simulink model "Fig237"  (R2014b)
settings: Solver=ode3  StartTime=0.0  StopTime=10  FixedStep=2e-5  RelTol=1e-5
libraries: commfilt2 x1, commchan3 x1, commsink2 x1, commrandsrc2 x1
settings Model: Creator=Dennis Silage  LastModifiedBy=Silage
settings DataIOCC: SignalLoggingSaveFormat=ModelDataLogs
settings OptimizationCC: ExpressionDepthLimit=2147483647  InitFltsAndDblsToZero=on
settings DebuggingCC: UnderspecifiedInitializationDetection=Classic  MergeDetectMultiDrivingBlocksExec=none  SolverPrmCheckMsg=none  FcnCallInpInsideContextMsg=UseLocalSettings  StateNameClashWarn=warning
settings GRTTargetCC: CombineOutputUpdateFcns=off  GRTInterface=on

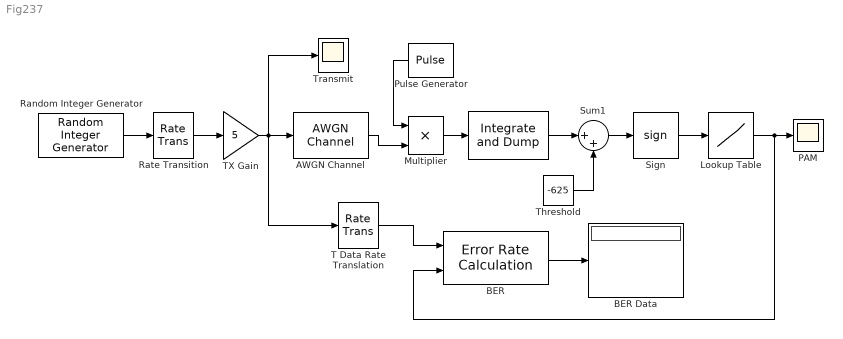
== system Fig237 ==
  " " : commfilt2/Integrate and Dump  obssamples=50  offsetsamples=0  nodump=off  roundingMode=Floor  overflowMode=off
  AWGN Channel : commchan3/AWGN Channel  InputProcessing=Inherited (this choice will be removed - see release notes)  seed=randseed  noiseMode="Signal to noise ratio  (Eb/No)"  EbNodB=40  EsNodB=10  SNRdB=10  bitsPerSym=1  Ps=25  Tsym=1e-3  variance=0
  BER : commsink2/Error Rate Calculation  N=1  st_delay=0  cp_mode=Entire frame  subframe=[]  PMode=Port  WsName=ErrorVec  RsMode2=off  stop=off  numErr=100  maxBits=1e6
  BER Data : Display
  Lookup Table : Lookup_n-D  NumberOfTableDimensions=1  BreakpointsForDimension1=[-1, 0, 1]  Table=[0, 0, 5]  InternalRulePriority=Speed  RndMeth=Nearest  InputSameDT=on
  Multiplier : Product  RndMeth=Zero
  PAM : Scope
      settings: TimeRange=0.05  YMin=-8  YMax=8
  Pulse Generator : DiscretePulseGenerator  PulseType=Time based  Amplitude=5  Period=1e-3  PulseWidth=98
  Random Integer Generator : commrandsrc2/Random Integer Generator  mul=2  seed=randseed  Ts=1e-3  frameBased=off  sampPerFrame=50  orient=on  outDataType=double
  Rate Transition : RateTransition  OutPortSampleTime=2e-5
  Sign : Signum
  Sum1 : Sum  Inputs=|++
  T Data Rate Translation : RateTransition  OutPortSampleTime=1e-3
  TX Gain : Gain  Gain=5
  Threshold : Constant  Value=-625
  Transmit : Scope
      settings: TimeRange=0.05  YMin=-8  YMax=8
  wires:
  TX Gain/1 -> T Data Rate Translation/1, Transmit/1, AWGN Channel/1
  Random Integer Generator/1 -> Rate Transition/1
  BER/1 -> BER Data/1
  T Data Rate Translation/1 -> BER/1
  Multiplier/1 -> " "/1
  AWGN Channel/1 -> Multiplier/2
  Pulse Generator/1 -> Multiplier/1
  Rate Transition/1 -> TX Gain/1
  Threshold/1 -> Sum1/2
  Sum1/1 -> Sign/1
  " "/1 -> Sum1/1
  Sign/1 -> Lookup Table/1
  Lookup Table/1 -> BER/2, PAM/1
